simulink model "predictive_continuous_simulation_20241118_2015b"  (R2015b)
settings: Solver=ode4  SolverMode=SingleTasking  StartTime=0.0  StopTime=Tend  FixedStep=Ts  MaxStep=Ts  MinStep=Ts  RelTol=1e-3
values from neighbouring files (symbols this model uses):
  gamma = 2    [code_simu.m]    (also in code_simu_continuous_simplified.m = 100000; matlab.mat = 1000)
  sigma = 10    [code_simu.m]    (also in code_simu_continuous_simplified.m = 0.01; matlab.mat = 100)
undefined symbols (not defined in the file or in its folder): ae, Afp, As, bap_bar, bap_v, be, beta0, beta1, beta2, bfp, cap_bar, den_filter, dena0, denf, denp, exp_cap2, fn, M1, M3, M3_v_2, M4_v_2, M_bar, num_filter, numa0, numf, nump, Pf, r, setpoint, setpoint_time, sin_f, T, T_gairan, Tf, Tf_n, Tf_n_vec, Tref, Ts, tstf_vec, v_max, YM
(part 1 of 2)
settings Model: Creator=IDS_PC  LastModifiedBy=IDS_PC
settings DataIOCC: LimitDataPoints=off
settings DebuggingCC: SolverPrmCheckMsg=warning  AllowSymbolicDim=on  StateNameClashWarn=warning  SFUnexpectedBacktrackingDiag=error  SFNoUnconditionalDefaultTransitionDiag=error
settings ModelReferenceCC: PropagateSignalLabelsOutOfModel=on
settings SFSimCC: SimUseLocalCustomCode=on
settings RTWCC: RTWUseLocalCustomCode=on
settings GRTTargetCC: TargetLangStandard=C99 (ISO)
settings ConfigComp: CovMetricSettings=dwe  CovSaveCumulativeToWorkspaceVar=off  CovSaveSingleToWorkspaceVar=off  CovModelRefEnable=Off  CovExternalEMLEnable=on

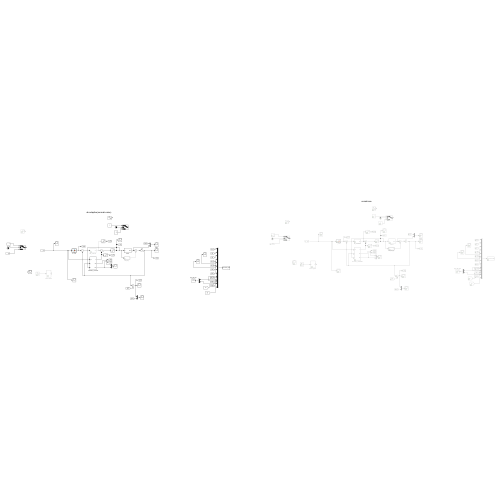
[thumbnail: Simulink's stored preview of the top-level diagram]
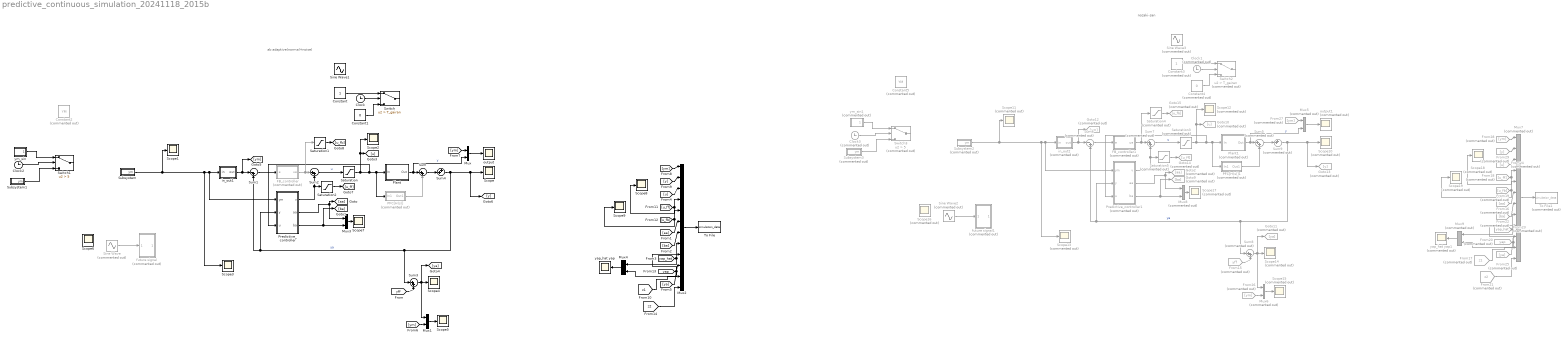
== system predictive_continuous_simulation_20241118_2015b ==
  note: ab adaptive(normal+noise)
  note: nozaki-san
  Clock : Clock
  Clock1 : Clock  Commented=on
  Clock2 : Clock
  Clock3 : Clock  Commented=on
  Constant : Constant
  Constant1 : Constant  Value=0
  Constant2 : Constant  Commented=on  Value=YM
  Constant3 : Constant  Commented=on
  Constant4 : Constant  Commented=on  Value=0
  Constant5 : Constant  Commented=on  Value=YM
  FB_controller : Subsystem  Commented=on
  FB_controller1 : Subsystem  Commented=on
  From15 : From  Commented=on  GotoTag=yff
  From16 : From  Commented=on  GotoTag=aa
  From17 : From  Commented=on  GotoTag=z1  TagVisibility=global
  From18 : From  Commented=on  GotoTag=u_ff
  From19 : From  Commented=on  GotoTag=u_fb
  From20 : From  Commented=on  GotoTag=yap  TagVisibility=global
  From21 : From  Commented=on  GotoTag=z2  TagVisibility=global
  From22 : From  Commented=on  GotoTag=ba
  From23 : From  Commented=on  GotoTag=yap_hat  TagVisibility=global
  From24 : From  Commented=on  GotoTag=u
  From25 : From  Commented=on  GotoTag=ya
  From26 : From  Commented=on  GotoTag=ym
  From27 : From  Commented=on  GotoTag=ym
  From28 : From  Commented=on  GotoTag=ym
  From29 : From  Commented=on  GotoTag=y
  Goto10 : Goto  Commented=on  GotoTag=u
  Goto11 : Goto  Commented=on  GotoTag=ya
  Goto12 : Goto  Commented=on  GotoTag=ym
  Goto13 : Goto  Commented=on  GotoTag=y
  Goto14 : Goto  Commented=on  GotoTag=u_ff
  Goto15 : Goto  Commented=on  GotoTag=u_fb
  Goto2 : Goto  Commented=on  GotoTag=aa
  Goto9 : Goto  Commented=on  GotoTag=ba
  Mux{,1,3..4} (4 alike) : Mux  Inputs=2
  Mux2 : Mux  Inputs=12
  Mux{5..6,8..9} (4 alike) : Mux  Commented=on  Inputs=2
  Mux7 : Mux  Commented=on  Inputs=12
  PFC[H(s)] : Subsystem  Commented=on  TreatAsAtomicUnit=on
  PFC[H(s)]1 : Subsystem  Commented=on  TreatAsAtomicUnit=on
  Plant : Subsystem
  Plant1 : Subsystem  Commented=on
  Predictive_controller : Subsystem
  Predictive_controller1 : Subsystem  Commented=on
  Saturation : Saturate  UpperLimit=v_max  LowerLimit=-v_max
  Saturation1 : Saturate  UpperLimit=v_max  LowerLimit=-v_max
  Saturation2 : Saturate  UpperLimit=v_max  LowerLimit=-v_max
  Saturation3 : Saturate  Commented=on  UpperLimit=v_max  LowerLimit=-v_max
  Saturation4 : Saturate  Commented=on  UpperLimit=v_max  LowerLimit=-v_max
  Saturation5 : Saturate  Commented=on  UpperLimit=v_max  LowerLimit=-v_max
  Scope{,1..9} (10 alike) : Scope
  Scope{10..19} (10 alike) : Scope  Commented=on
  Sine Wave : Sin  Commented=on  Frequency=2*pi*fn  SampleTime=0
  Sine Wave1 : Sin  Amplitude=0.1  Frequency=2*pi*1  SampleTime=0
  Sine Wave2 : Sin  Commented=on  Frequency=2*pi*fn  SampleTime=0
  Sine Wave3 : Sin  Commented=on  Amplitude=0.1  Frequency=2*pi*1  SampleTime=0
  Subsystem : Subsystem
  Subsystem1 : Subsystem
  Subsystem2 : Subsystem  Commented=on
  Subsystem3 : Subsystem  Commented=on
  Sum : Sum  Inputs=|++
  Sum1 : Sum  Inputs=|-+
  Sum2 : Sum  Inputs=|++
  Sum3 : Sum  Inputs=|++
  Sum4 : Sum  Inputs=++|
  Sum5 : Sum  Commented=on  Inputs=|++
  Sum6 : Sum  Commented=on  Inputs=|-+
  Sum7 : Sum  Commented=on  Inputs=|++
  Sum8 : Sum  Commented=on  Inputs=|++
  Sum9 : Sum  Commented=on  Inputs=++|
  Switch : Switch  Criteria=u2 > Threshold  Threshold=T_gairan
  Switch1 : Switch  Criteria=u2 > Threshold  Threshold=5
  Switch2 : Switch  Commented=on  Criteria=u2 > Threshold  Threshold=T_gairan
  Switch3 : Switch  Commented=on  Criteria=u2 > Threshold  Threshold=5
  To File : ToFile  Filename=simulation_data
  To File1 : ToFile  Commented=on  Filename=simulation_data
  future signal : Subsystem  Commented=on
  future signal1 : Subsystem  Commented=on
  in_out1 : MATLAB Function  TreatAsAtomicUnit=on
  in_out2 : MATLAB Function  Commented=on  TreatAsAtomicUnit=on
  output : Scope
  output1 : Scope  Commented=on
  yap_hat yap : Scope
  yap_hat yap1 : Scope  Commented=on
  ym_sin : Subsystem
  ym_sin1 : Subsystem  Commented=on
  wires:
  [y] -> Mux2/2
  Mux4/1 -> yap_hat yap/1
  [ym] -> Mux/1
  [yap_hat] -> Mux4/1, Mux2/8
  Mux3/1 -> Scope7/1
  Sine Wave/1 -> future signal/1(In1)
  Constant1/1 -> Switch/3
  Constant/1 -> Switch/1
  Predictive_controller/1(v) -> Saturation2/1, Sum2/2
  [u_ff] -> Scope8/1, Mux2/4
  [u] -> Mux2/3
  [yap] -> Mux4/2, Mux2/9
  [ym] -> Mux1/2
  Saturation/1 -> [u], Scope2/1, PFC[H(s)]/1(In1), Plant/1(In), Predictive_controller/3(u)
  [ym] -> Mux2/1
  [u_fb] -> Scope9/1, Mux2/5
  Saturation1/1 -> [u_fb]
  Mux1/1 -> Scope5/1
  [aa] -> Mux2/6
  Sum3/1 -> [ya], Mux1/1, Scope4/1
  Predictive_controller/3(ba) -> Mux3/2, [ba]
  Plant/1(Out) -> Mux/2, Sum/1  "y"
  Predictive_controller/2(aa) -> [aa], Mux3/1
  Subsystem/1(ym) -> Scope1/1, Predictive_controller/1(ym), in_out1/1(in), Scope3/1
  Clock/1 -> Switch/2
  [ba] -> Mux2/7
  [yff] -> Sum3/2
  [ya] -> Mux2/10
  Sum4/1 -> [y], Scope/1, Predictive_controller/2(y), Sum1/2, Sum3/1  "ya"
  Mux/1 -> output/1
  Mux2/1 -> To File/1
  Sum1/1 -> FB_controller/1(e)
  Sum2/1 -> Saturation/1  "u"
  Saturation2/1 -> [u_ff]
  FB_controller/1(ue) -> Saturation1/1, Sum2/1
  PFC[H(s)]/1(Out1) -> Sum/2
  Sum/1 -> Sum4/2
  in_out1/1(out) -> [ym], Sum1/1
  Clock2/1 -> Switch1/2
  ym_sin/1(Out1) -> Switch1/1
  Subsystem1/1(ym) -> Switch1/3
  [z1] -> Mux2/11
  [z2] -> Mux2/12
  From21/1 -> Mux7/12
  Subsystem3/1(ym) -> Switch3/3
  Saturation4/1 -> Goto15/1
  From25/1 -> Mux7/10
  Mux8/1 -> Scope17/1
  From20/1 -> Mux9/2, Mux7/9
  ym_sin1/1(Out1) -> Switch3/1
  From22/1 -> Mux7/7
  in_out2/1(out) -> Goto12/1, Sum6/1
  FB_controller1/1(ue) -> Saturation4/1, Sum7/1
  Predictive_controller1/1(v) -> Saturation5/1, Sum7/2
  Saturation5/1 -> Goto14/1
  Clock3/1 -> Switch3/2
  Sum7/1 -> Saturation3/1  "u"
  Plant1/1(Out) -> Mux5/2, Sum5/1  "y"
  From29/1 -> Mux7/2
  Sum6/1 -> FB_controller1/1(e)
  Mux5/1 -> output1/1
  Mux6/1 -> Scope15/1
  PFC[H(s)]1/1(Out1) -> Sum5/2
  From27/1 -> Mux5/1
  Subsystem2/1(ym) -> Scope11/1, Predictive_controller1/1(ym), in_out2/1(in), Scope13/1
  From18/1 -> Scope18/1, Mux7/4
  Clock1/1 -> Switch2/2
  Sum8/1 -> Goto11/1, Mux6/1, Scope14/1
  Saturation3/1 -> Goto10/1, Scope12/1, PFC[H(s)]1/1(In1), Plant1/1(In), Predictive_controller1/3(u)
  Constant3/1 -> Switch2/1
  Predictive_controller1/2(aa) -> Goto2/1, Mux8/1
  From19/1 -> Scope19/1, Mux7/5
  Sum9/1 -> Goto13/1, Scope10/1, Predictive_controller1/2(y), Sum6/2, Sum8/1  "ya"
  From24/1 -> Mux7/3
  From15/1 -> Sum8/2
  Mux7/1 -> To File1/1
  From16/1 -> Mux7/6
  From23/1 -> Mux9/1, Mux7/8
  From17/1 -> Mux7/11
  Predictive_controller1/3(ba) -> Mux8/2, Goto9/1
  From28/1 -> Mux7/1
  Sum5/1 -> Sum9/2
  From26/1 -> Mux6/2
  Mux9/1 -> yap_hat yap1/1
  Sine Wave2/1 -> future signal1/1(In1)
  Constant4/1 -> Switch2/3

== system predictive_continuous_simulation_20241118_2015b/FB_controller ==
  e : Inport
  FB_controller : Subsystem
  PFC : TransferFcn  Numerator=numa0  Denominator=dena0
  Scope : Scope
  Sum : Sum  Inputs=|++
  ue : Outport
  tag scope: yff=global
  wires:
  e/1 -> Sum/1
  PFC/1 -> [yff], Scope/1
  Sum/1 -> FB_controller/1(eaf)
  FB_controller/1(ue) -> ue/1
  ? -> PFC/1

== system predictive_continuous_simulation_20241118_2015b/FB_controller1 ==
  e : Inport
  FB_controller : Subsystem
  PFC : TransferFcn  Numerator=numa0  Denominator=dena0
  Scope : Scope
  Sum : Sum  Inputs=|++
  ue : Outport
  tag scope: yff=global
  wires:
  e/1 -> Sum/1
  PFC/1 -> [yff], Scope/1
  Sum/1 -> FB_controller/1(eaf)
  FB_controller/1(ue) -> ue/1
  ? -> PFC/1

== system predictive_continuous_simulation_20241118_2015b/PFC[H(s)] ==
  In1 : Inport
  F(s) : TransferFcn  Numerator=numf  Denominator=denf
  G0(s) : TransferFcn  Numerator=numa0  Denominator=dena0
  Sum : Sum  Inputs=|+-
  Sum1 : Sum  Inputs=|++
  Transport Delay : TransportDelay  DelayTime=T
  Out1 : Outport
  wires:
  In1/1 -> F(s)/1, Sum/1, Transport Delay/1
  G0(s)/1 -> Sum1/1
  Transport Delay/1 -> Sum/2
  Sum/1 -> G0(s)/1
  Sum1/1 -> Out1/1
  F(s)/1 -> Sum1/2

== system predictive_continuous_simulation_20241118_2015b/PFC[H(s)]1 ==
  In1 : Inport
  F(s) : TransferFcn  Numerator=numf  Denominator=denf
  G0(s) : TransferFcn  Numerator=numa0  Denominator=dena0
  Sum : Sum  Inputs=|+-
  Sum1 : Sum  Inputs=|++
  Transport Delay : TransportDelay  DelayTime=T
  Out1 : Outport
  wires:
  In1/1 -> F(s)/1, Sum/1, Transport Delay/1
  G0(s)/1 -> Sum1/1
  Transport Delay/1 -> Sum/2
  Sum/1 -> G0(s)/1
  Sum1/1 -> Out1/1
  F(s)/1 -> Sum1/2

== system predictive_continuous_simulation_20241118_2015b/Plant ==
  In : Inport
  Transfer Fcn : TransferFcn  Numerator=nump  Denominator=denp
  Transport Delay : TransportDelay  DelayTime=T
  Out : Outport
  wires:
  Transfer Fcn/1 -> Out/1
  In/1 -> Transport Delay/1
  Transport Delay/1 -> Transfer Fcn/1

== system predictive_continuous_simulation_20241118_2015b/Plant1 ==
  In : Inport
  Transfer Fcn : TransferFcn  Numerator=nump  Denominator=denp
  Transport Delay : TransportDelay  DelayTime=T
  Out : Outport
  wires:
  Transfer Fcn/1 -> Out/1
  In/1 -> Transport Delay/1
  Transport Delay/1 -> Transfer Fcn/1

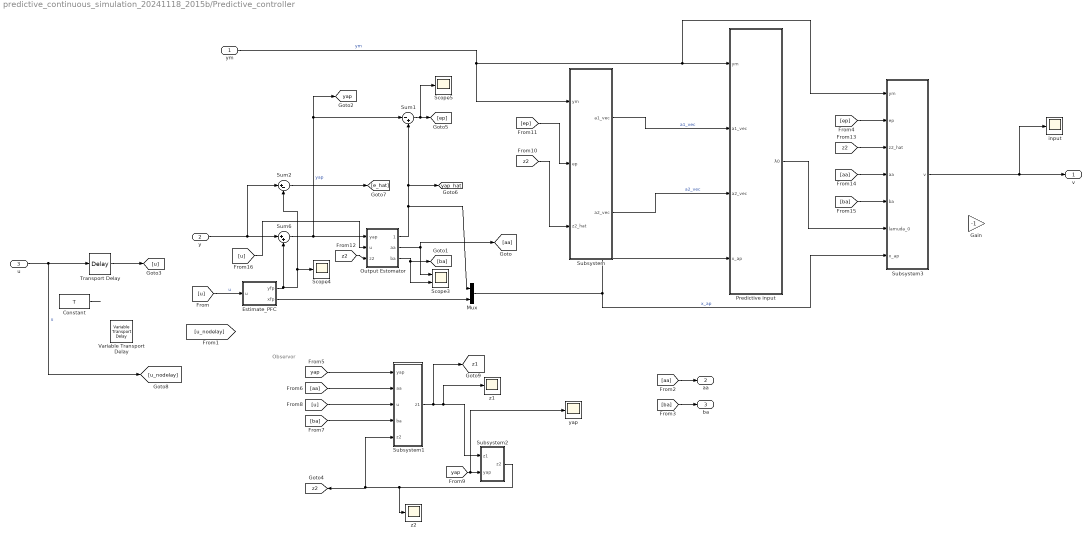
== system predictive_continuous_simulation_20241118_2015b/Predictive_controller ==
  note: Observor
  ym : Inport
  y : Inport  Port=2
  u : Inport  Port=3
  Constant : Constant  Value=T
  Estimate_PFC : Subsystem
  Gain : Gain  Gain=-1
  Mux : Mux  Inputs=2
  Output Estomator : Subsystem
  Predictive input : Subsystem
  Scope3 : Scope  NumInputPorts=2
  Scope4 : Scope
  Scope5 : Scope
  Subsystem : Subsystem
  Subsystem1 : Subsystem
  Subsystem2 : Subsystem
  Subsystem3 : Subsystem
  Sum1 : Sum  Inputs=|-+
  Sum2 : Sum  Inputs=|+-
  Sum6 : Sum  Inputs=|++
  Transport Delay : TransportDelay  DelayTime=T
  Variable Transport Delay : VariableTransportDelay  MaximumDelay=10
  input : Scope
  yap : Scope
  z1 : Scope
  z2 : Scope
  v : Outport
  aa : Outport  Port=2
  ba : Outport  Port=3
  tag scope: yap=global, yap_hat=global, z1=global, z2=global
  wires:
  y/1 -> Sum2/1, Sum6/1
  Estimate_PFC/1(yfp) -> Scope4/1, Sum2/2, Sum6/2
  Sum6/1 -> Sum1/1, [yap], Output Estomator/1(yap)  "yap"
  Output Estomator/1(yap_hat) -> Mux/1, [yap_hat], Sum1/2
  Estimate_PFC/2(xfp) -> Mux/2
  ym/1 -> Subsystem/1(ym), Subsystem3/1(ym), Predictive input/1(ym)  "ym"
  Mux/1 -> Predictive input/4(x_ap), Subsystem3/7(x_ap)  "x_ap"
  Subsystem/2(a2_vec) -> Predictive input/3(a2_vec)  "a2_vec"
  Subsystem/1(a1_vec) -> Predictive input/2(a1_vec)  "a1_vec"
  u/1 -> Transport Delay/1, [u_nodelay]  "u"
  [z2] -> Subsystem/3(z2_hat)
  Output Estomator/2(aa) -> [aa], Scope3/1
  Output Estomator/3(ba) -> [ba], Scope3/2
  [aa] -> aa/1
  [ba] -> ba/1
  [yap] -> Subsystem1/1(yap)
  [aa] -> Subsystem1/2(aa)
  [u] -> Subsystem1/3(u)
  [ba] -> Subsystem1/4("ba ")
  Subsystem2/1(z2) -> z2/1, Subsystem1/5(z2), [z2]
  Sum1/1 -> Scope5/1, [ep]
  [ep] -> Subsystem/2(ep)
  [z2] -> Output Estomator/3("z2 ")
  Sum2/1 -> [e_hat]
  Predictive input/1(λ0) -> Subsystem3/6("lamuda_0 ")
  [ba] -> Subsystem3/5(ba)
  [aa] -> Subsystem3/4(aa)
  [z2] -> Subsystem3/3(z2_hat)
  [ep] -> Subsystem3/2(ep)
  [u] -> Estimate_PFC/1(u)  "u"
  [u] -> Output Estomator/2(u)
  Constant/1 -> ?
  [yap] -> yap/1, Subsystem2/2(yap)
  Transport Delay/1 -> [u]
  Subsystem3/1(v) -> input/1, v/1
  Subsystem1/1(z1) -> [z1], z1/1, Subsystem2/1(z1)

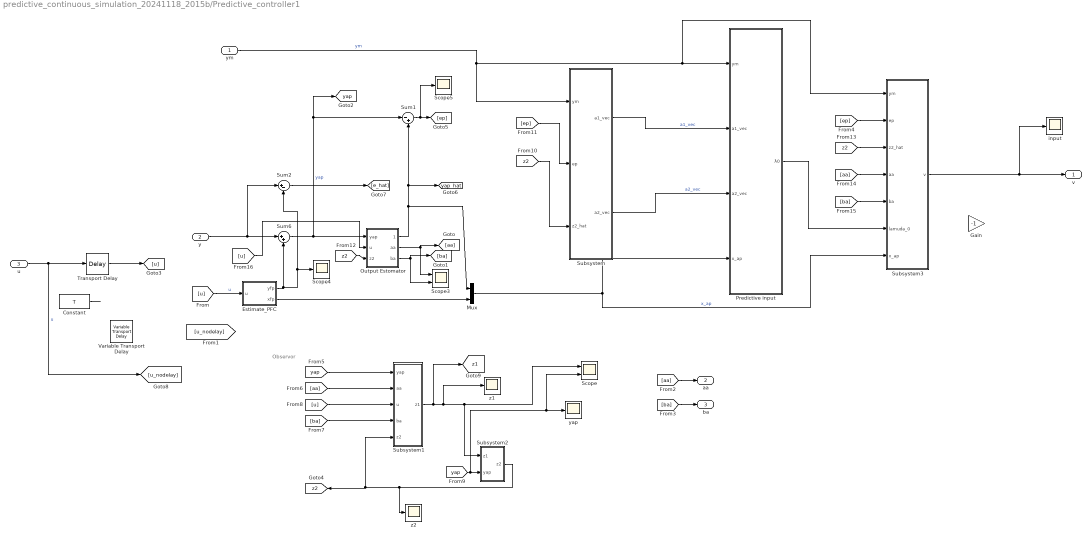
== system predictive_continuous_simulation_20241118_2015b/Predictive_controller1 ==
  note: Observor
  ym : Inport
  y : Inport  Port=2
  u : Inport  Port=3
  Constant : Constant  Value=T
  Estimate_PFC : Subsystem
  Gain : Gain  Gain=-1
  Mux : Mux  Inputs=2
  Output Estomator : Subsystem
  Predictive input : Subsystem
  Scope : Scope  NumInputPorts=2
  Scope3 : Scope  NumInputPorts=2
  Scope4 : Scope
  Scope5 : Scope
  Subsystem : Subsystem
  Subsystem1 : Subsystem
  Subsystem2 : Subsystem
  Subsystem3 : Subsystem
  Sum1 : Sum  Inputs=|-+
  Sum2 : Sum  Inputs=|+-
  Sum6 : Sum  Inputs=|++
  Transport Delay : TransportDelay  DelayTime=T
  Variable Transport Delay : VariableTransportDelay  MaximumDelay=10
  input : Scope
  yap : Scope
  z1 : Scope
  z2 : Scope
  v : Outport
  aa : Outport  Port=2
  ba : Outport  Port=3
  tag scope: yap=global, yap_hat=global, z1=global, z2=global
  wires:
  y/1 -> Sum2/1, Sum6/1
  Estimate_PFC/1(yfp) -> Scope4/1, Sum2/2, Sum6/2
  Sum6/1 -> Sum1/1, [yap], Output Estomator/1(yap)  "yap"
  Output Estomator/1(yap_hat) -> Mux/1, [yap_hat], Sum1/2
  Estimate_PFC/2(xfp) -> Mux/2
  ym/1 -> Subsystem/1(ym), Subsystem3/1(ym), Predictive input/1(ym)  "ym"
  Mux/1 -> Predictive input/4(x_ap), Subsystem3/7(x_ap)  "x_ap"
  Subsystem/2(a2_vec) -> Predictive input/3(a2_vec)  "a2_vec"
  Subsystem/1(a1_vec) -> Predictive input/2(a1_vec)  "a1_vec"
  u/1 -> Transport Delay/1, [u_nodelay]  "u"
  [z2] -> Subsystem/3(z2_hat)
  Output Estomator/2(aa) -> [aa], Scope3/1
  Output Estomator/3(ba) -> [ba], Scope3/2
  [aa] -> aa/1
  [ba] -> ba/1
  [yap] -> Subsystem1/1(yap)
  [aa] -> Subsystem1/2(aa)
  [u] -> Subsystem1/3(u)
  [ba] -> Subsystem1/4("ba ")
  Subsystem2/1(z2) -> z2/1, Subsystem1/5(z2), [z2]
  Sum1/1 -> Scope5/1, [ep]
  [ep] -> Subsystem/2(ep)
  [z2] -> Output Estomator/3("z2 ")
  Sum2/1 -> [e_hat]
  Predictive input/1(λ0) -> Subsystem3/6("lamuda_0 ")
  [ba] -> Subsystem3/5(ba)
  [aa] -> Subsystem3/4(aa)
  [z2] -> Subsystem3/3(z2_hat)
  [ep] -> Subsystem3/2(ep)
  [u] -> Estimate_PFC/1(u)  "u"
  [u] -> Output Estomator/2(u)
  Constant/1 -> ?
  [yap] -> Scope/2, yap/1, Subsystem2/2(yap)
  Subsystem3/1(v) -> input/1, v/1
  Subsystem1/1(z1) -> Scope/1, Subsystem2/1(z1), z1/1, [z1]
  Transport Delay/1 -> [u]

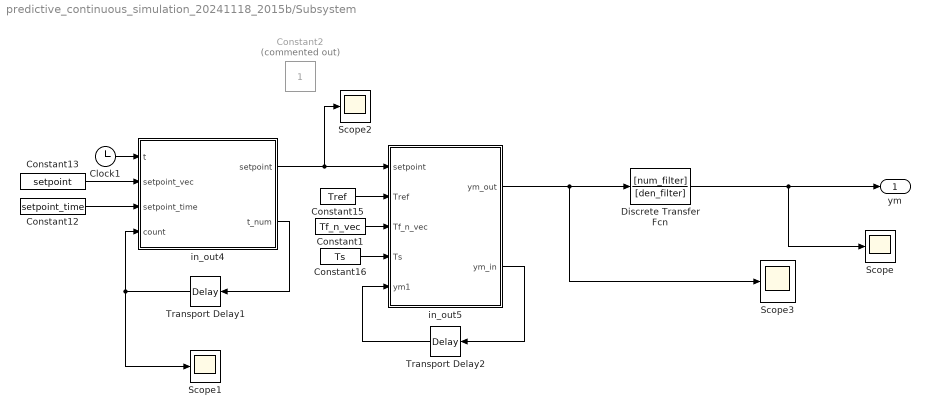
== system predictive_continuous_simulation_20241118_2015b/Subsystem ==
  Clock1 : Clock
  Constant1 : Constant  Value=Tf_n_vec
  Constant12 : Constant  Value=setpoint_time
  Constant13 : Constant  Value=setpoint
  Constant15 : Constant  Value=Tref
  Constant16 : Constant  Value=Ts
  Constant2 : Constant  Commented=on
  Discrete Transfer Fcn : DiscreteTransferFcn  Numerator=[num_filter]  Denominator=[den_filter]
  Scope{,1..3} (4 alike) : Scope
  Transport Delay1 : TransportDelay  DelayTime=Ts  InitialOutput=1
  Transport Delay2 : TransportDelay  DelayTime=Ts
  in_out4 : MATLAB Function  TreatAsAtomicUnit=on
  in_out5 : MATLAB Function  TreatAsAtomicUnit=on
  ym : Outport
  wires:
  Constant12/1 -> in_out4/3(setpoint_time)
  in_out4/2(t_num) -> Transport Delay1/1
  Transport Delay1/1 -> Scope1/1, in_out4/4(count)
  Constant13/1 -> in_out4/2(setpoint_vec)
  Constant15/1 -> in_out5/2(Tref)
  Constant16/1 -> in_out5/4(Ts)
  Transport Delay2/1 -> in_out5/5(ym1)
  in_out5/2(ym_in) -> Transport Delay2/1
  Constant1/1 -> in_out5/3(Tf_n_vec)
  Clock1/1 -> in_out4/1(t)
  in_out4/1(setpoint) -> Scope2/1, in_out5/1(setpoint)
  in_out5/1(ym_out) -> Discrete Transfer Fcn/1, Scope3/1
  Discrete Transfer Fcn/1 -> Scope/1, ym/1

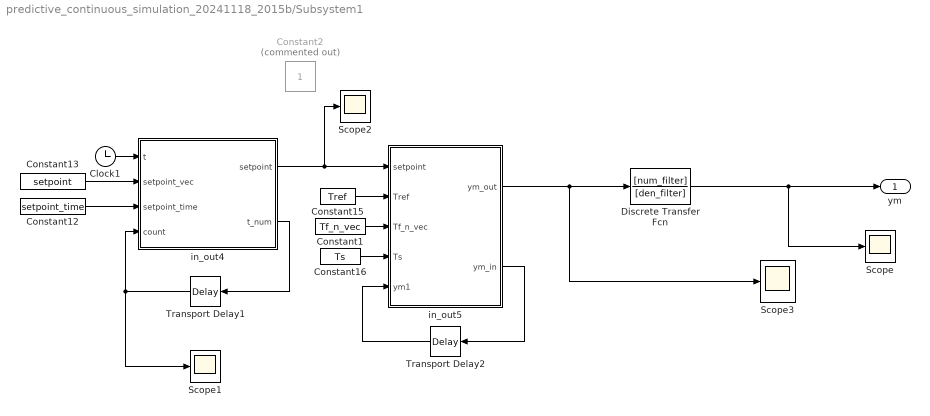
== system predictive_continuous_simulation_20241118_2015b/Subsystem1 ==
  Clock1 : Clock
  Constant1 : Constant  Value=Tf_n_vec
  Constant12 : Constant  Value=setpoint_time
  Constant13 : Constant  Value=setpoint
  Constant15 : Constant  Value=Tref
  Constant16 : Constant  Value=Ts
  Constant2 : Constant  Commented=on
  Discrete Transfer Fcn : DiscreteTransferFcn  Numerator=[num_filter]  Denominator=[den_filter]
  Scope{,1..3} (4 alike) : Scope
  Transport Delay1 : TransportDelay  DelayTime=Ts  InitialOutput=1
  Transport Delay2 : TransportDelay  DelayTime=Ts
  in_out4 : MATLAB Function  TreatAsAtomicUnit=on
  in_out5 : MATLAB Function  TreatAsAtomicUnit=on
  ym : Outport
  wires:
  Discrete Transfer Fcn/1 -> ym/1, Scope/1
  in_out5/1(ym_out) -> Scope3/1, Discrete Transfer Fcn/1
  in_out4/1(setpoint) -> in_out5/1(setpoint), Scope2/1
  Clock1/1 -> in_out4/1(t)
  Constant1/1 -> in_out5/3(Tf_n_vec)
  in_out5/2(ym_in) -> Transport Delay2/1
  Transport Delay2/1 -> in_out5/5(ym1)
  Constant16/1 -> in_out5/4(Ts)
  Constant15/1 -> in_out5/2(Tref)
  Constant13/1 -> in_out4/2(setpoint_vec)
  Transport Delay1/1 -> in_out4/4(count), Scope1/1
  in_out4/2(t_num) -> Transport Delay1/1
  Constant12/1 -> in_out4/3(setpoint_time)

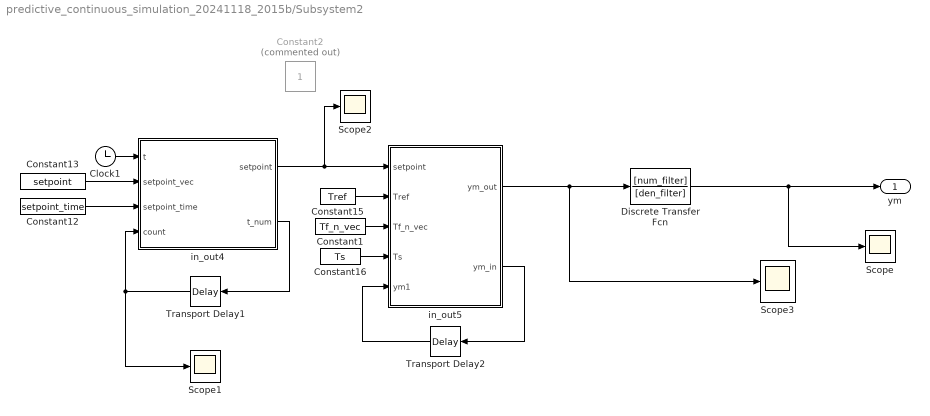
== system predictive_continuous_simulation_20241118_2015b/Subsystem2 ==
  Clock1 : Clock
  Constant1 : Constant  Value=Tf_n_vec
  Constant12 : Constant  Value=setpoint_time
  Constant13 : Constant  Value=setpoint
  Constant15 : Constant  Value=Tref
  Constant16 : Constant  Value=Ts
  Constant2 : Constant  Commented=on
  Discrete Transfer Fcn : DiscreteTransferFcn  Numerator=[num_filter]  Denominator=[den_filter]
  Scope{,1..3} (4 alike) : Scope
  Transport Delay1 : TransportDelay  DelayTime=Ts  InitialOutput=1
  Transport Delay2 : TransportDelay  DelayTime=Ts
  in_out4 : MATLAB Function  TreatAsAtomicUnit=on
  in_out5 : MATLAB Function  TreatAsAtomicUnit=on
  ym : Outport
  wires:
  Constant12/1 -> in_out4/3(setpoint_time)
  in_out4/2(t_num) -> Transport Delay1/1
  Transport Delay1/1 -> Scope1/1, in_out4/4(count)
  Constant13/1 -> in_out4/2(setpoint_vec)
  Constant15/1 -> in_out5/2(Tref)
  Constant16/1 -> in_out5/4(Ts)
  Transport Delay2/1 -> in_out5/5(ym1)
  in_out5/2(ym_in) -> Transport Delay2/1
  Constant1/1 -> in_out5/3(Tf_n_vec)
  Clock1/1 -> in_out4/1(t)
  in_out4/1(setpoint) -> Scope2/1, in_out5/1(setpoint)
  in_out5/1(ym_out) -> Discrete Transfer Fcn/1, Scope3/1
  Discrete Transfer Fcn/1 -> Scope/1, ym/1

== system predictive_continuous_simulation_20241118_2015b/Subsystem3 ==
  Clock1 : Clock
  Constant1 : Constant  Value=Tf_n_vec
  Constant12 : Constant  Value=setpoint_time
  Constant13 : Constant  Value=setpoint
  Constant15 : Constant  Value=Tref
  Constant16 : Constant  Value=Ts
  Constant2 : Constant  Commented=on
  Discrete Transfer Fcn : DiscreteTransferFcn  Numerator=[num_filter]  Denominator=[den_filter]
  Scope{,1..3} (4 alike) : Scope
  Transport Delay1 : TransportDelay  DelayTime=Ts  InitialOutput=1
  Transport Delay2 : TransportDelay  DelayTime=Ts
  in_out4 : MATLAB Function  TreatAsAtomicUnit=on
  in_out5 : MATLAB Function  TreatAsAtomicUnit=on
  ym : Outport
  wires:
  Discrete Transfer Fcn/1 -> ym/1, Scope/1
  in_out5/1(ym_out) -> Scope3/1, Discrete Transfer Fcn/1
  in_out4/1(setpoint) -> in_out5/1(setpoint), Scope2/1
  Clock1/1 -> in_out4/1(t)
  Constant1/1 -> in_out5/3(Tf_n_vec)
  in_out5/2(ym_in) -> Transport Delay2/1
  Transport Delay2/1 -> in_out5/5(ym1)
  Constant16/1 -> in_out5/4(Ts)
  Constant15/1 -> in_out5/2(Tref)
  Constant13/1 -> in_out4/2(setpoint_vec)
  Transport Delay1/1 -> in_out4/4(count), Scope1/1
  in_out4/2(t_num) -> Transport Delay1/1
  Constant12/1 -> in_out4/3(setpoint_time)

== system predictive_continuous_simulation_20241118_2015b/future signal ==
  In1 : Inport
  Constant : Constant  Value=Tf_n_vec
  Constant1 : Constant  Value=0
  Constant2 : Constant
  MATLAB Function : MATLAB Function  TreatAsAtomicUnit=on
  Switch : Switch  Criteria=u2 > Threshold  Threshold=0.5
  Transport Delay1 : TransportDelay  DelayTime=Ts
  Transport Delay2 : TransportDelay  DelayTime=Ts*Tf_n
  Out1 : Outport
  wires:
  In1/1 -> MATLAB Function/1(u)
  Transport Delay1/1 -> MATLAB Function/3(u_in)
  MATLAB Function/1(ym) -> Switch/1, Transport Delay1/1
  Constant/1 -> MATLAB Function/2(Tf_n_vec)
  Constant1/1 -> Switch/3
  Constant2/1 -> Transport Delay2/1
  Transport Delay2/1 -> Switch/2
  Switch/1 -> Out1/1

== system predictive_continuous_simulation_20241118_2015b/future signal1 ==
  In1 : Inport
  Constant : Constant  Value=Tf_n_vec
  Constant1 : Constant  Value=0
  Constant2 : Constant
  MATLAB Function : MATLAB Function  TreatAsAtomicUnit=on
  Switch : Switch  Criteria=u2 > Threshold  Threshold=0.5
  Transport Delay1 : TransportDelay  DelayTime=Ts
  Transport Delay2 : TransportDelay  DelayTime=Ts*Tf_n
  Out1 : Outport
  wires:
  In1/1 -> MATLAB Function/1(u)
  Transport Delay1/1 -> MATLAB Function/3(u_in)
  MATLAB Function/1(ym) -> Switch/1, Transport Delay1/1
  Constant/1 -> MATLAB Function/2(Tf_n_vec)
  Constant1/1 -> Switch/3
  Constant2/1 -> Transport Delay2/1
  Transport Delay2/1 -> Switch/2
  Switch/1 -> Out1/1

== system predictive_continuous_simulation_20241118_2015b/ym_sin ==
  Constant1 : Constant  Value=sin_f
  Constant2 : Constant  Value=Tf_n_vec
  Constant3 : Constant  Value=Ts
  Constant4 : Constant  Value=Ts
  MATLAB Function : MATLAB Function  TreatAsAtomicUnit=on
  Product : Product
  Scope : Scope
  Scope1 : Scope
  Step : Step  Time=Ts  SampleTime=0
  Sum : Sum  Inputs=|++
  Transport Delay : TransportDelay  DelayTime=Ts
  Transport Delay1 : TransportDelay  DelayTime=5
  Out1 : Outport
  wires:
  Product/1 -> Sum/1
  MATLAB Function/1(ym) -> Transport Delay1/1
  Constant2/1 -> MATLAB Function/1(Tf_n_vec)
  Constant3/1 -> MATLAB Function/3(Ts)
  Constant1/1 -> MATLAB Function/4(omega_sin)
  Constant4/1 -> Product/1
  Step/1 -> Product/2
  Sum/1 -> Scope1/1, Transport Delay/1, MATLAB Function/2(t)
  Transport Delay/1 -> Sum/2
  Transport Delay1/1 -> Scope/1, Out1/1

== system predictive_continuous_simulation_20241118_2015b/ym_sin1 ==
  Constant1 : Constant  Value=sin_f
  Constant2 : Constant  Value=Tf_n_vec
  Constant3 : Constant  Value=Ts
  Constant4 : Constant  Value=Ts
  MATLAB Function : MATLAB Function  TreatAsAtomicUnit=on
  Product : Product
  Scope : Scope
  Scope1 : Scope
  Step : Step  Time=Ts  SampleTime=0
  Sum : Sum  Inputs=|++
  Transport Delay : TransportDelay  DelayTime=Ts
  Transport Delay1 : TransportDelay  DelayTime=5
  Out1 : Outport
  wires:
  Product/1 -> Sum/1
  MATLAB Function/1(ym) -> Transport Delay1/1
  Constant2/1 -> MATLAB Function/1(Tf_n_vec)
  Constant3/1 -> MATLAB Function/3(Ts)
  Constant1/1 -> MATLAB Function/4(omega_sin)
  Constant4/1 -> Product/1
  Step/1 -> Product/2
  Sum/1 -> Scope1/1, Transport Delay/1, MATLAB Function/2(t)
  Transport Delay/1 -> Sum/2
  Transport Delay1/1 -> Scope/1, Out1/1

== system predictive_continuous_simulation_20241118_2015b/FB_controller/FB_controller ==
  eaf : Inport
  Gain : Gain  Gain=-1
  Integrator : Integrator
  Math Function : Math  Operator=square  SaturateOnIntegerOverflow=on
  Product : Product
  Product1 : Product
  Product2 : Product
  Scope : Scope
  Sum1 : Sum  Inputs=|++
  To Workspace : ToWorkspace  VariableName=theta_vec  SampleTime=-1
  γ : Constant  Value=gamma
  σ : Constant  Value=sigma
  ue : Outport
  wires:
  Math Function/1 -> Product1/1
  γ/1 -> Product1/2
  eaf/1 -> Product/1, Math Function/1
  Product1/1 -> Sum1/1
  Product2/1 -> Sum1/2
  Sum1/1 -> Integrator/1
  σ/1 -> Product2/1
  Integrator/1 -> To Workspace/1, Scope/1, Gain/1, Product2/2  "θ"
  Gain/1 -> Product/2
  Product/1 -> ue/1

== system predictive_continuous_simulation_20241118_2015b/FB_controller1/FB_controller ==
  eaf : Inport
  Gain : Gain  Gain=-1
  Integrator : Integrator
  Math Function : Math  Operator=square  SaturateOnIntegerOverflow=on
  Product : Product
  Product1 : Product
  Product2 : Product
  Scope : Scope
  Sum1 : Sum  Inputs=|++
  To Workspace : ToWorkspace  VariableName=theta_vec  SampleTime=-1
  γ : Constant  Value=gamma
  σ : Constant  Value=sigma
  ue : Outport
  wires:
  Math Function/1 -> Product1/1
  γ/1 -> Product1/2
  eaf/1 -> Product/1, Math Function/1
  Product1/1 -> Sum1/1
  Product2/1 -> Sum1/2
  Sum1/1 -> Integrator/1
  σ/1 -> Product2/1
  Integrator/1 -> To Workspace/1, Scope/1, Gain/1, Product2/2  "θ"
  Gain/1 -> Product/2
  Product/1 -> ue/1

== system predictive_continuous_simulation_20241118_2015b/Predictive_controller/Estimate_PFC ==
  u : Inport
  Gain : Gain  Gain=bfp  Multiplication=Matrix(K*u)
  Gain1 : Gain  Gain=Afp  Multiplication=Matrix(K*u) (u vector)
  Gain2 : Gain  Gain=cfp.'  Multiplication=Matrix(K*u) (u vector)
  Integrator : Integrator
  Scope : Scope
  Sum2 : Sum  Inputs=|++
  yfp : Outport
  xfp : Outport  Port=2
  wires:
  u/1 -> Gain/1
  Sum2/1 -> Integrator/1
  Gain/1 -> Sum2/1  "b_fp*u"
  Integrator/1 -> xfp/1, Gain2/1, Gain1/1  "x_fp"
  Gain1/1 -> Sum2/2
  Gain2/1 -> Scope/1, yfp/1

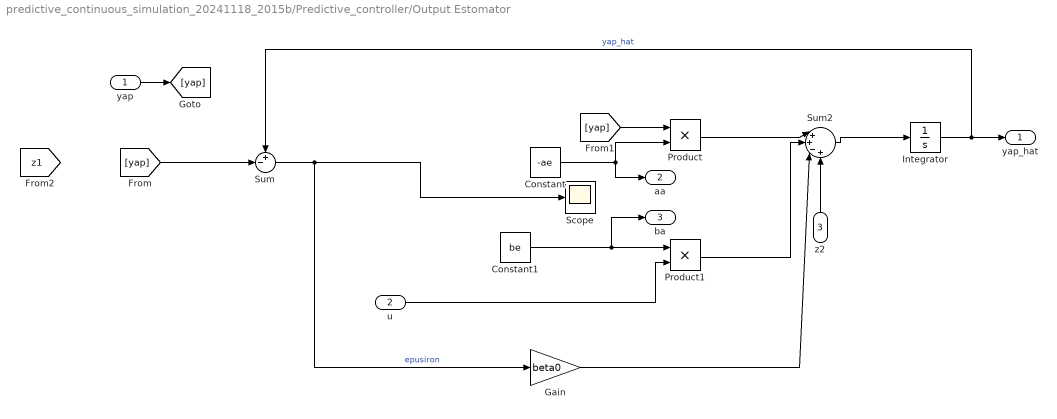
== system predictive_continuous_simulation_20241118_2015b/Predictive_controller/Output Estomator ==
  yap : Inport
  u : Inport  Port=2
  "z2 " : Inport  Port=3
  Constant : Constant  Value=-ae
  Constant1 : Constant  Value=be
  Gain : Gain  Gain=beta0
  Integrator : Integrator
  Product : Product
  Product1 : Product
  Scope : Scope
  Sum : Sum  Inputs=+-|
  Sum2 : Sum  Inputs=|++-+
  yap_hat : Outport
  aa : Outport  Port=2
  ba : Outport  Port=3
  wires:
  Sum/1 -> Gain/1, Scope/1  "epusiron"
  Product1/1 -> Sum2/2
  Sum2/1 -> Integrator/1
  Product/1 -> Sum2/1
  [yap] -> Sum/2
  u/1 -> Product1/2
  Constant/1 -> aa/1, Product/2
  Constant1/1 -> ba/1, Product1/1
  Integrator/1 -> Sum/1, yap_hat/1  "yap_hat"
  Gain/1 -> Sum2/3
  "z2 "/1 -> Sum2/4
  yap/1 -> [yap]
  [yap] -> Product/1

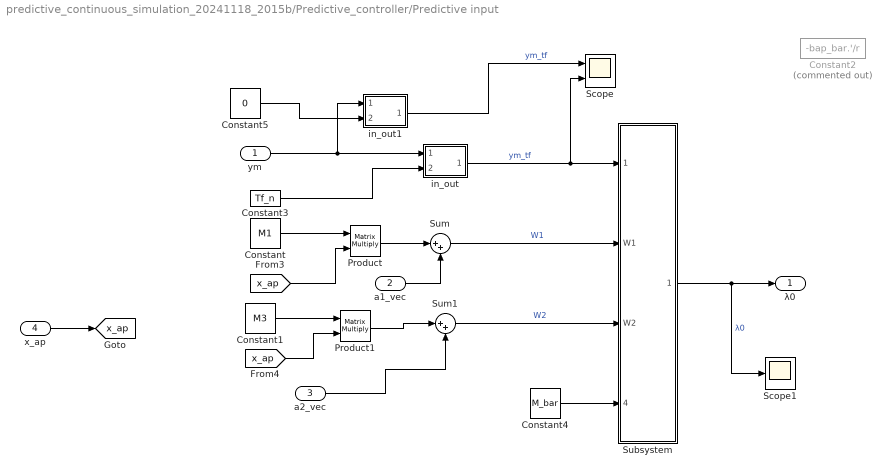
== system predictive_continuous_simulation_20241118_2015b/Predictive_controller/Predictive input ==
  ym : Inport
  a1_vec : Inport  Port=2
  a2_vec : Inport  Port=3
  x_ap : Inport  Port=4
  Constant : Constant  Value=M1
  Constant1 : Constant  Value=M3
  Constant2 : Constant  Commented=on  Value=-bap_bar.'/r  VectorParams1D=off  SampleTime=-1
  Constant3 : Constant  Value=Tf_n
  Constant4 : Constant  Value=M_bar
  Constant5 : Constant  Value=0
  Product : Product  Multiplication=Matrix(*)
  Product1 : Product  Multiplication=Matrix(*)
  Scope : Scope  NumInputPorts=2
  Scope1 : Scope
  Subsystem : Subsystem
  Sum : Sum  Inputs=|++
  Sum1 : Sum  Inputs=|++
  in_out : MATLAB Function  TreatAsAtomicUnit=on
  in_out1 : MATLAB Function  TreatAsAtomicUnit=on
  λ0 : Outport
  tag scope: x_ap=global
  wires:
  x_ap/1 -> [x_ap]
  Constant/1 -> Product/1
  [x_ap] -> Product/2
  Product/1 -> Sum/1
  a1_vec/1 -> Sum/2
  Constant1/1 -> Product1/1
  [x_ap] -> Product1/2
  Product1/1 -> Sum1/1
  a2_vec/1 -> Sum1/2
  ym/1 -> in_out1/1(ym_vec), in_out/1(ym_vec)
  in_out/1(ym_tf) -> Scope/2, Subsystem/1(ym_tf)  "ym_tf"
  Sum1/1 -> Subsystem/3(W2)  "W2"
  Sum/1 -> Subsystem/2(W1)  "W1"
  Constant3/1 -> in_out/2(Tf_n)
  Constant4/1 -> Subsystem/4(M_bar)
  Subsystem/1(lambda_0) -> Scope1/1, λ0/1  "λ0"
  Constant5/1 -> in_out1/2(Tf_n)
  in_out1/1(ym_tf) -> Scope/1  "ym_tf"

== system predictive_continuous_simulation_20241118_2015b/Predictive_controller/Subsystem ==
  ym : Inport
  ep : Inport  Port=2
  z2_hat : Inport  Port=3
  Constant : Constant  Value=cap_bar
  Constant2 : Constant  Value=beta0
  Constant3 : Constant  Value=Tf_n
  Constant4 : Constant  Value=Ts
  Constant5 : Constant  Value=Tf
  Constant6 : Constant  Value=tstf_vec
  MATLAB Function1 : MATLAB Function  TreatAsAtomicUnit=on
  a1_vec : Outport
  a2_vec : Outport  Port=2
  wires:
  ym/1 -> MATLAB Function1/1(ym)
  ep/1 -> MATLAB Function1/2(ep)
  z2_hat/1 -> MATLAB Function1/3(z2_hat)
  Constant/1 -> MATLAB Function1/4(cap_bar)
  Constant2/1 -> MATLAB Function1/5(beta0)
  MATLAB Function1/2(a2_vec) -> a2_vec/1
  MATLAB Function1/1(a1_vec) -> a1_vec/1
  Constant3/1 -> MATLAB Function1/6(Tf_n)
  Constant4/1 -> MATLAB Function1/7(Ts)
  Constant5/1 -> MATLAB Function1/8(Tf)
  Constant6/1 -> MATLAB Function1/9(tstf_vec)

== system predictive_continuous_simulation_20241118_2015b/Predictive_controller/Subsystem1 ==
  yap : Inport
  aa : Inport  Port=2
  u : Inport  Port=3
  "ba " : Inport  Port=4
  z2 : Inport  Port=5
  Gain : Gain  Gain=-beta1
  Integrator : Integrator
  Product : Product
  Product1 : Product
  Sum2 : Sum  Inputs=|++
  Sum3 : Sum  Inputs=-+|
  Sum4 : Sum  Inputs=++|
  Sum5 : Sum  Inputs=|++
  z1 : Outport
  wires:
  Sum2/1 -> Sum4/2
  u/1 -> Product1/1
  Product/1 -> Sum2/1
  yap/1 -> Sum3/1
  Sum4/1 -> Sum5/1
  Gain/1 -> Sum4/1
  Product1/1 -> Sum2/2
  Integrator/1 -> z1/1, Product/1, Sum3/2
  z2/1 -> Sum5/2
  "ba "/1 -> Product1/2
  Sum5/1 -> Integrator/1
  Sum3/1 -> Gain/1
  aa/1 -> Product/2

== system predictive_continuous_simulation_20241118_2015b/Predictive_controller/Subsystem2 ==
  z1 : Inport
  yap : Inport  Port=2
  Gain1 : Gain  Gain=-beta2
  Integrator1 : Integrator
  Sum7 : Sum  Inputs=+-|
  z2 : Outport
  wires:
  yap/1 -> Sum7/2
  Sum7/1 -> Gain1/1
  Integrator1/1 -> z2/1
  z1/1 -> Sum7/1
  Gain1/1 -> Integrator1/1

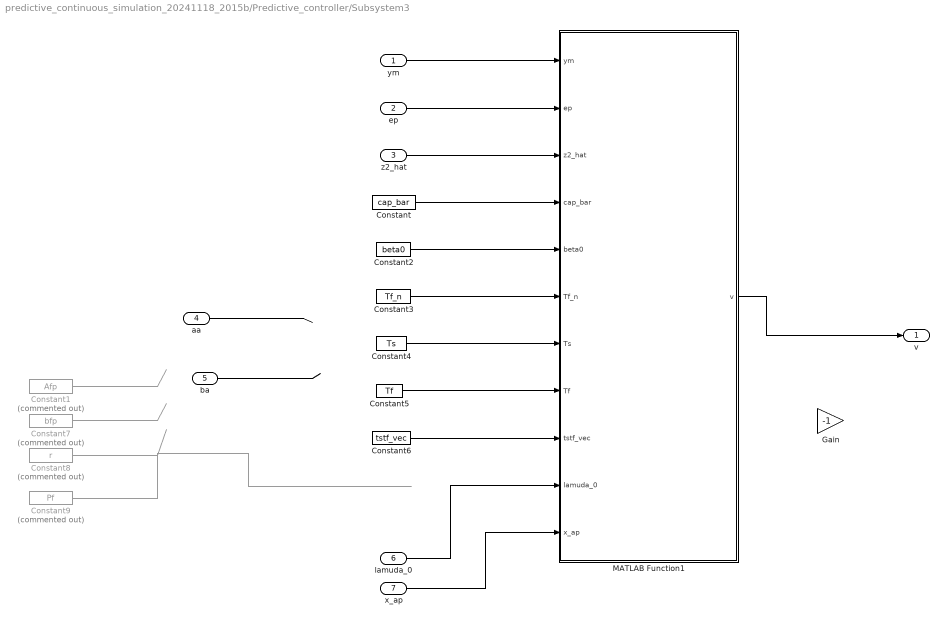
== system predictive_continuous_simulation_20241118_2015b/Predictive_controller/Subsystem3 ==
  ym : Inport
  ep : Inport  Port=2
  z2_hat : Inport  Port=3
  aa : Inport  Port=4
  ba : Inport  Port=5
  "lamuda_0 " : Inport  Port=6
  x_ap : Inport  Port=7
  Constant : Constant  Value=cap_bar
  Constant1 : Constant  Commented=on  Value=Afp
  Constant2 : Constant  Value=beta0
  Constant3 : Constant  Value=Tf_n
  Constant4 : Constant  Value=Ts
  Constant5 : Constant  Value=Tf
  Constant6 : Constant  Value=tstf_vec
  Constant7 : Constant  Commented=on  Value=bfp
  Constant8 : Constant  Commented=on  Value=r
  Constant9 : Constant  Commented=on  Value=Pf
  Gain : Gain  Gain=-1
  MATLAB Function1 : MATLAB Function  TreatAsAtomicUnit=on
      settings: MinAlgLoopOccurrences=on
  v : Outport
  wires:
  ym/1 -> MATLAB Function1/1(ym)
  ep/1 -> MATLAB Function1/2(ep)
  z2_hat/1 -> MATLAB Function1/3(z2_hat)
  Constant/1 -> MATLAB Function1/4(cap_bar)
  Constant2/1 -> MATLAB Function1/5(beta0)
  Constant3/1 -> MATLAB Function1/6(Tf_n)
  Constant4/1 -> MATLAB Function1/7(Ts)
  Constant5/1 -> MATLAB Function1/8(Tf)
  Constant6/1 -> MATLAB Function1/9(tstf_vec)
  aa/1 -> ?
  ba/1 -> ?
  Constant1/1 -> ?
  Constant7/1 -> ?
  Constant8/1 -> ?
  Constant9/1 -> ?
  "lamuda_0 "/1 -> MATLAB Function1/10(lamuda_0)
  x_ap/1 -> MATLAB Function1/11(x_ap)
  MATLAB Function1/1(v) -> v/1

== system predictive_continuous_simulation_20241118_2015b/Predictive_controller1/Estimate_PFC ==
  u : Inport
  Gain : Gain  Gain=bfp  Multiplication=Matrix(K*u)
  Gain1 : Gain  Gain=Afp  Multiplication=Matrix(K*u) (u vector)
  Gain2 : Gain  Gain=cfp.'  Multiplication=Matrix(K*u) (u vector)
  Integrator : Integrator
  Scope : Scope
  Sum2 : Sum  Inputs=|++
  yfp : Outport
  xfp : Outport  Port=2
  wires:
  u/1 -> Gain/1
  Sum2/1 -> Integrator/1
  Gain/1 -> Sum2/1  "b_fp*u"
  Integrator/1 -> xfp/1, Gain2/1, Gain1/1  "x_fp"
  Gain1/1 -> Sum2/2
  Gain2/1 -> Scope/1, yfp/1

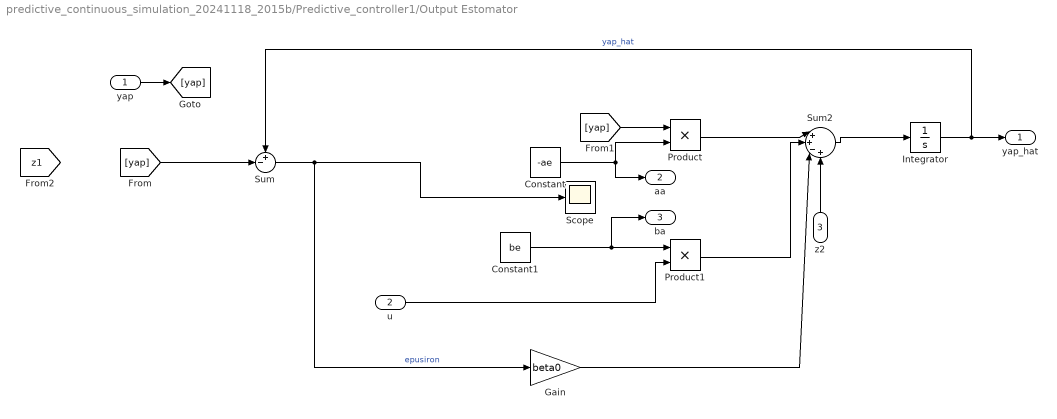
== system predictive_continuous_simulation_20241118_2015b/Predictive_controller1/Output Estomator ==
  yap : Inport
  u : Inport  Port=2
  "z2 " : Inport  Port=3
  Constant : Constant  Value=-ae
  Constant1 : Constant  Value=be
  Gain : Gain  Gain=beta0
  Integrator : Integrator
  Product : Product
  Product1 : Product
  Scope : Scope
  Sum : Sum  Inputs=+-|
  Sum2 : Sum  Inputs=|++-+
  yap_hat : Outport
  aa : Outport  Port=2
  ba : Outport  Port=3
  wires:
  Sum/1 -> Gain/1, Scope/1  "epusiron"
  Product1/1 -> Sum2/2
  Sum2/1 -> Integrator/1
  Product/1 -> Sum2/1
  [yap] -> Sum/2
  u/1 -> Product1/2
  Constant/1 -> aa/1, Product/2
  Constant1/1 -> ba/1, Product1/1
  Integrator/1 -> Sum/1, yap_hat/1  "yap_hat"
  Gain/1 -> Sum2/3
  "z2 "/1 -> Sum2/4
  yap/1 -> [yap]
  [yap] -> Product/1

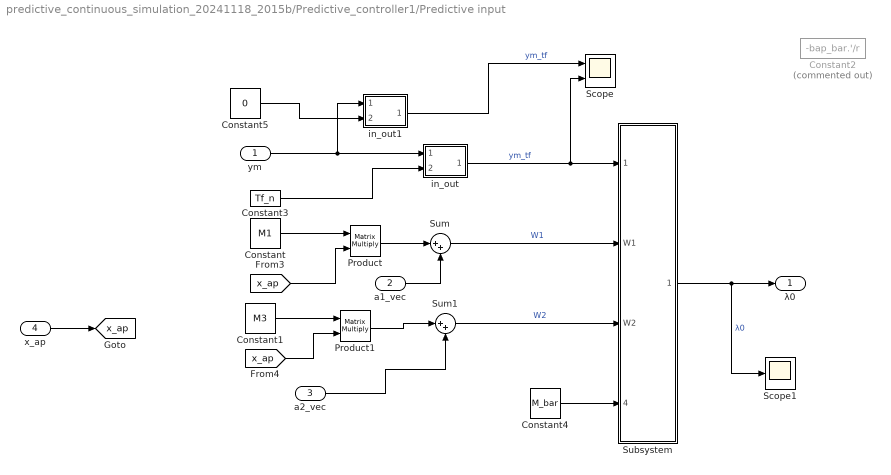
== system predictive_continuous_simulation_20241118_2015b/Predictive_controller1/Predictive input ==
  ym : Inport
  a1_vec : Inport  Port=2
  a2_vec : Inport  Port=3
  x_ap : Inport  Port=4
  Constant : Constant  Value=M1
  Constant1 : Constant  Value=M3
  Constant2 : Constant  Commented=on  Value=-bap_bar.'/r  VectorParams1D=off  SampleTime=-1
  Constant3 : Constant  Value=Tf_n
  Constant4 : Constant  Value=M_bar
  Constant5 : Constant  Value=0
  Product : Product  Multiplication=Matrix(*)
  Product1 : Product  Multiplication=Matrix(*)
  Scope : Scope  NumInputPorts=2
  Scope1 : Scope
  Subsystem : Subsystem
  Sum : Sum  Inputs=|++
  Sum1 : Sum  Inputs=|++
  in_out : MATLAB Function  TreatAsAtomicUnit=on
  in_out1 : MATLAB Function  TreatAsAtomicUnit=on
  λ0 : Outport
  tag scope: x_ap=global
  wires:
  x_ap/1 -> [x_ap]
  Constant/1 -> Product/1
  [x_ap] -> Product/2
  Product/1 -> Sum/1
  a1_vec/1 -> Sum/2
  Constant1/1 -> Product1/1
  [x_ap] -> Product1/2
  Product1/1 -> Sum1/1
  a2_vec/1 -> Sum1/2
  ym/1 -> in_out1/1(ym_vec), in_out/1(ym_vec)
  in_out/1(ym_tf) -> Scope/2, Subsystem/1(ym_tf)  "ym_tf"
  Sum1/1 -> Subsystem/3(W2)  "W2"
  Sum/1 -> Subsystem/2(W1)  "W1"
  Constant3/1 -> in_out/2(Tf_n)
  Constant4/1 -> Subsystem/4(M_bar)
  Subsystem/1(lambda_0) -> Scope1/1, λ0/1  "λ0"
  Constant5/1 -> in_out1/2(Tf_n)
  in_out1/1(ym_tf) -> Scope/1  "ym_tf"

== system predictive_continuous_simulation_20241118_2015b/Predictive_controller1/Subsystem ==
  ym : Inport
  ep : Inport  Port=2
  z2_hat : Inport  Port=3
  Constant : Constant  Value=cap_bar
  Constant2 : Constant  Value=beta0
  Constant3 : Constant  Value=Tf_n
  Constant4 : Constant  Value=Ts
  Constant5 : Constant  Value=Tf
  Constant6 : Constant  Value=tstf_vec
  MATLAB Function1 : MATLAB Function  TreatAsAtomicUnit=on
  a1_vec : Outport
  a2_vec : Outport  Port=2
  wires:
  ym/1 -> MATLAB Function1/1(ym)
  ep/1 -> MATLAB Function1/2(ep)
  z2_hat/1 -> MATLAB Function1/3(z2_hat)
  Constant/1 -> MATLAB Function1/4(cap_bar)
  Constant2/1 -> MATLAB Function1/5(beta0)
  MATLAB Function1/2(a2_vec) -> a2_vec/1
  MATLAB Function1/1(a1_vec) -> a1_vec/1
  Constant3/1 -> MATLAB Function1/6(Tf_n)
  Constant4/1 -> MATLAB Function1/7(Ts)
  Constant5/1 -> MATLAB Function1/8(Tf)
  Constant6/1 -> MATLAB Function1/9(tstf_vec)

== system predictive_continuous_simulation_20241118_2015b/Predictive_controller1/Subsystem1 ==
  yap : Inport
  aa : Inport  Port=2
  u : Inport  Port=3
  "ba " : Inport  Port=4
  z2 : Inport  Port=5
  Gain : Gain  Gain=-beta1
  Integrator : Integrator
  Product : Product
  Product1 : Product
  Sum2 : Sum  Inputs=|++
  Sum3 : Sum  Inputs=-+|
  Sum4 : Sum  Inputs=++|
  Sum5 : Sum  Inputs=|++
  z1 : Outport
  wires:
  Sum2/1 -> Sum4/2
  u/1 -> Product1/1
  Product/1 -> Sum2/1
  yap/1 -> Sum3/1
  Sum4/1 -> Sum5/1
  Gain/1 -> Sum4/1
  Product1/1 -> Sum2/2
  Integrator/1 -> z1/1, Product/1, Sum3/2
  z2/1 -> Sum5/2
  "ba "/1 -> Product1/2
  Sum5/1 -> Integrator/1
  Sum3/1 -> Gain/1
  aa/1 -> Product/2

== system predictive_continuous_simulation_20241118_2015b/Predictive_controller1/Subsystem2 ==
  z1 : Inport
  yap : Inport  Port=2
  Gain1 : Gain  Gain=-beta2
  Integrator1 : Integrator
  Sum7 : Sum  Inputs=+-|
  z2 : Outport
  wires:
  yap/1 -> Sum7/2
  Sum7/1 -> Gain1/1
  Integrator1/1 -> z2/1
  z1/1 -> Sum7/1
  Gain1/1 -> Integrator1/1

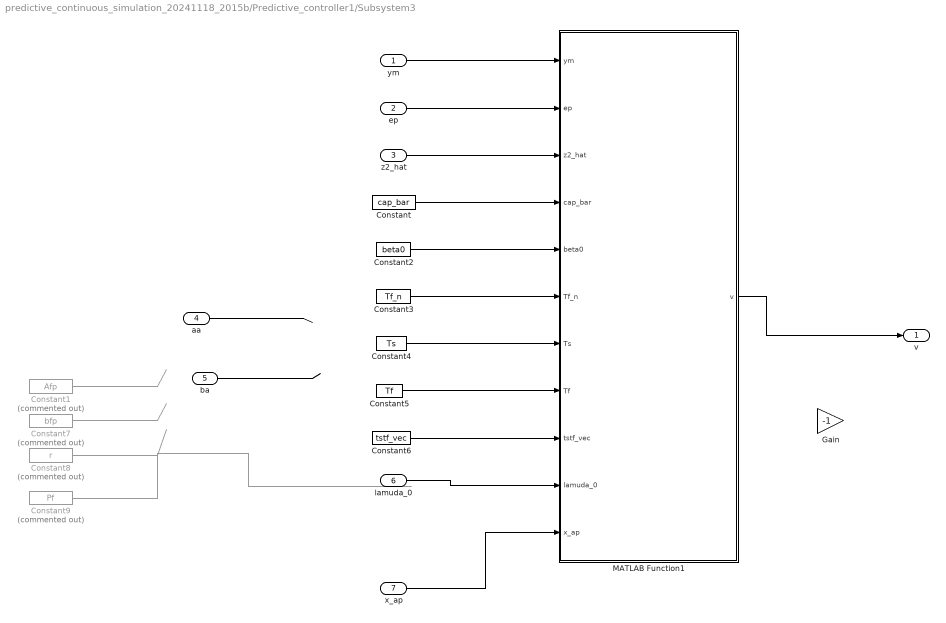
== system predictive_continuous_simulation_20241118_2015b/Predictive_controller1/Subsystem3 ==
  ym : Inport
  ep : Inport  Port=2
  z2_hat : Inport  Port=3
  aa : Inport  Port=4
  ba : Inport  Port=5
  "lamuda_0 " : Inport  Port=6
  x_ap : Inport  Port=7
  Constant : Constant  Value=cap_bar
  Constant1 : Constant  Commented=on  Value=Afp
  Constant2 : Constant  Value=beta0
  Constant3 : Constant  Value=Tf_n
  Constant4 : Constant  Value=Ts
  Constant5 : Constant  Value=Tf
  Constant6 : Constant  Value=tstf_vec
  Constant7 : Constant  Commented=on  Value=bfp
  Constant8 : Constant  Commented=on  Value=r
  Constant9 : Constant  Commented=on  Value=Pf
  Gain : Gain  Gain=-1
  MATLAB Function1 : MATLAB Function  TreatAsAtomicUnit=on
      settings: MinAlgLoopOccurrences=on
  v : Outport
  wires:
  ym/1 -> MATLAB Function1/1(ym)
  ep/1 -> MATLAB Function1/2(ep)
  z2_hat/1 -> MATLAB Function1/3(z2_hat)
  Constant/1 -> MATLAB Function1/4(cap_bar)
  Constant2/1 -> MATLAB Function1/5(beta0)
  Constant3/1 -> MATLAB Function1/6(Tf_n)
  Constant4/1 -> MATLAB Function1/7(Ts)
  Constant5/1 -> MATLAB Function1/8(Tf)
  Constant6/1 -> MATLAB Function1/9(tstf_vec)
  aa/1 -> ?
  ba/1 -> ?
  Constant1/1 -> ?
  Constant7/1 -> ?
  Constant8/1 -> ?
  Constant9/1 -> ?
  "lamuda_0 "/1 -> MATLAB Function1/10(lamuda_0)
  x_ap/1 -> MATLAB Function1/11(x_ap)
  MATLAB Function1/1(v) -> v/1

== system predictive_continuous_simulation_20241118_2015b/Predictive_controller/Predictive input/Subsystem ==
  ym_tf : Inport
  W1 : Inport  Port=2
  W2 : Inport  Port=3
  M_bar : Inport  Port=4
  Constant : Constant  Value=Pf
  Constant1 : Constant  Value=cap_bar
  MATLAB Function : MATLAB Function  TreatAsAtomicUnit=on
  lambda_0 : Outport
  wires:
  ym_tf/1 -> MATLAB Function/1(ym_tf)
  W1/1 -> MATLAB Function/2(W1)
  W2/1 -> MATLAB Function/3(W2)
  Constant/1 -> MATLAB Function/4(Pf)
  Constant1/1 -> MATLAB Function/5(cap_bar)
  MATLAB Function/1(lambda_0) -> lambda_0/1
  M_bar/1 -> MATLAB Function/6(M_bar)

== system predictive_continuous_simulation_20241118_2015b/Predictive_controller1/Predictive input/Subsystem ==
  ym_tf : Inport
  W1 : Inport  Port=2
  W2 : Inport  Port=3
  M_bar : Inport  Port=4
  Constant : Constant  Value=Pf
  Constant1 : Constant  Value=cap_bar
  MATLAB Function : MATLAB Function  TreatAsAtomicUnit=on
  lambda_0 : Outport
  wires:
  ym_tf/1 -> MATLAB Function/1(ym_tf)
  W1/1 -> MATLAB Function/2(W1)
  W2/1 -> MATLAB Function/3(W2)
  Constant/1 -> MATLAB Function/4(Pf)
  Constant1/1 -> MATLAB Function/5(cap_bar)
  MATLAB Function/1(lambda_0) -> lambda_0/1
  M_bar/1 -> MATLAB Function/6(M_bar)

== matlab function predictive_continuous_simulation_20241118_2015b/Subsystem/in_out4 ==
  data: setpoint output; t input; setpoint_vec input; t_num output; setpoint_time input; count input
function [setpoint,t_num]  = fcn(t,setpoint_vec,setpoint_time,count)
%#codegen
%%% 目標値の生成

count_n = count;

if(count_n<=length(setpoint_time) && t>=setpoint_time(int8(count_n)) && t~=0)
    count_n = count_n+1;
end

setpoint = setpoint_vec(int8(count_n));

t_num = count_n;

== matlab function predictive_continuous_simulation_20241118_2015b/Predictive_controller/Predictive input/Subsystem/MATLAB Function ==
  data: ym_tf input; W1 input; W2 input; lambda_0 output; Pf input; cap_bar input; M_bar input
function lambda_0  = fcn(ym_tf,W1,W2,Pf,cap_bar,M_bar)
%#codegen
Wq=ones(4,1);
Wq=W1;

%%% [λ(t0) ν_f]^T の計算
    lambda_nu = M_bar*[Pf*Wq-W2;ym_tf-cap_bar.'*Wq];

    
    lambda_0 = lambda_nu(1:length(lambda_nu)-1,1);  % λ(t0)
%     nu = lambda_nu(length(lambda_nu),:);            % ν_f

== matlab function predictive_continuous_simulation_20241118_2015b/Predictive_controller/Predictive input/in_out ==
  data: ym_vec input; ym_tf output; Tf_n input
function ym_tf = fcn(ym_vec,Tf_n)

% nym=zeros(Tf_n+1,1);
% nym=ym_vec;
%#codegen
ym_tf = ym_vec(1,Tf_n+1);
% ym_tf = nym(Tf_n+1,1);

== matlab function predictive_continuous_simulation_20241118_2015b/ym_sin/MATLAB Function ==
  data: Tf_n_vec input; ym output; t input; Ts input; omega_sin input
function ym = fcn(Tf_n_vec,t,Ts,omega_sin)
a = length(Tf_n_vec)+1

ym = zeros(1,a)
for i = 1:a
    ym(i) = sin(2*pi*omega_sin*(t+(i-1)*Ts))+0.5;
end

== matlab function predictive_continuous_simulation_20241118_2015b/Predictive_controller/Subsystem/MATLAB Function1 ==
  data: ym input; ep input; z2_hat input; a1_vec output; a2_vec output; cap_bar input; beta0 input; Tf_n input; Ts input; Tf input; tstf_vec input; As parameter; exp_cap2 parameter
function [a1_vec,a2_vec] = fcn(ym,ep,z2_hat,cap_bar,beta0,Tf_n,Ts,Tf,tstf_vec,As,exp_cap2)
%#codegen
% % aa,ba,Afp,bfp,r,Pf
%     Aap_bar = [aa zeros(1,length(Afp)); zeros(length(Afp),1) Afp];
%     bap_bar = [ba;bfp];
%     As = [Aap_bar -bap_bar*bap_bar.'/r; -cap_bar*cap_bar.' -Aap_bar.'];
%     
%     M = expm(As*(Tf));                    
%     M1 = M(1:length(M)/2 , 1:length(M)/2);
%     M2 = M(1:length(M)/2 , length(M)/2+1:length(M));
%     M3 = M(length(M)/2+1:length(M) , 1:length(M)/2);
%     M4 = M(length(M)/2+1:length(M) , length(M)/2+1:length(M));
%     
%     M_bar = inv([M4-Pf*M2 -cap_bar; cap_bar.'*M2 0]);
%     
%     bap_v = -bap_bar.'/r;     % ****** %

 %%%--------------------------------------------------------------------%%
 %%%--------------------------------------------------------------------%%
 
a_vec = zeros(length(cap_bar)*2,length(tstf_vec));
a_vec_int = zeros(length(cap_bar)*2,1);

%%%  tf-t0
%%% ∫     exp(As*tau)*tr([0 ca_bar])*ym(tf-tau)*dtau
%%%  0
%%% 台形積分を使用
%%% サンプリング時間ごとの，0からtf-t0までの被積分関数値を計算 
    ii=1;
    for i = 0:Ts:Tf
%         a_vec(:,round(1+i/Ts)) = expm(As*i)*[[1;zeros(length(cap_bar)-1,1)] zeros(length(cap_bar),1); zeros(length(cap_bar),1) cap_bar]*[z2_hat-beta0*ep;ym(round(Tf_n+1-i/Ts))]; 
        a_vec(:,round(1+i/Ts)) = exp_cap2(:,:,ii)*[z2_hat-beta0*ep;ym(round(Tf_n+1-i/Ts))];
%         a_vec(:,round(1+i/Ts)) = exp_cap2(:,:,ii)*[z2_hat;ym(1,round(Tf_n+1-i/Ts))];
        ii=ii+1;
    end
%%% 台形積分
    for i = 1:length(As)
        a_vec_int(i,1) = trapz(tstf_vec,a_vec(i,:));
    end

        a1_vec = a_vec_int(1:length(cap_bar));
        a2_vec = a_vec_int(length(cap_bar)+1:length(cap_bar)*2);

== matlab function predictive_continuous_simulation_20241118_2015b/future signal/MATLAB Function ==
  data: u input; Tf_n_vec input; ym output; u_in input
function ym = fcn(u,Tf_n_vec,u_in)


a = length(Tf_n_vec);
ym = zeros(1,a + 1);
ym(1,1:a) = u_in(1,2:a+1);
ym(1,a+1) = u;

== matlab function predictive_continuous_simulation_20241118_2015b/Subsystem/in_out5 ==
  data: setpoint input; Tref input; Tf_n_vec input; Ts input; ym_out output; ym1 input; ym_in output
function [ym_out,ym_in]   = fcn(setpoint,Tref,Tf_n_vec,Ts,ym1)
%#codegen
%%% 規範信号の生成
%%% 現時刻:ym(t) から 現時刻＋予測時間:ym(t+Tf) まで

nym = length(Tf_n_vec)+1;

ym = zeros(1,nym);
ym(1) = ym1;
    for k = 2:nym
        ym(1,k) = setpoint - exp(-Ts/Tref)*(setpoint-ym(1,k-1));
    end
ym_out = ym;
ym_in = ym(2);

== matlab function predictive_continuous_simulation_20241118_2015b/in_out1 ==
  data: in input; out output
function out = fcn(in)
%#codegen
out = in(1,1);

== matlab function predictive_continuous_simulation_20241118_2015b/Predictive_controller/Subsystem3/MATLAB Function1 ==
  data: ym input; ep input; z2_hat input; v output; cap_bar input; beta0 input; Tf_n input; Ts input; Tf input; tstf_vec input; lamuda_0 input; x_ap input; M3_v_2 parameter; M4_v_2 parameter; As parameter; bap_v parameter; T parameter; exp_cap2 parameter
function v = fcn(ym,ep,z2_hat,cap_bar,beta0,Tf_n,Ts,Tf,tstf_vec,lamuda_0,x_ap,M3_v_2, M4_v_2,As,bap_v,T,exp_cap2)
%#codegen
% aa,ba,Afp,bfp,r,Pf,T
%     Aap_bar = [aa zeros(1,length(Afp)); zeros(length(Afp),1) Afp];
%     bap_bar = [ba;bfp];
%     As = [Aap_bar -bap_bar*bap_bar.'/r; -cap_bar*cap_bar.' -Aap_bar.'];
% 
% M3_v = zeros(length(As)/2,length(As)/2,length(tstf_vec));
% M4_v = zeros(length(As)/2,length(As)/2,length(tstf_vec));
%   for j = 0:Ts:Tf 
%     M = expm(As*(j));                    
% %     M1 = M(1:length(M)/2 , 1:length(M)/2);
% %     M2 = M(1:length(M)/2 , length(M)/2+1:length(M));
%     M3 = M(length(M)/2+1:length(M) , 1:length(M)/2);
%     M4 = M(length(M)/2+1:length(M) , length(M)/2+1:length(M));
%     
%     M3_v(:,:,round(1+j/Ts)) = M3;
%     M4_v(:,:,round(1+j/Ts)) = M4;
%     
%     % M_bar = inv([M4-Pf*M2 -cap_bar; cap_bar.'*M2 0]);  
%     
%         
%   end
%   bap_v = -bap_bar.'/r; 
 %%%--------------------------------------------------------------------%%
 %%%--------------------------------------------------------------------%%
 
a_vec = zeros(length(cap_bar)*2,length(tstf_vec));
a_vec_int = zeros(length(cap_bar)*2,1);

%%%  tf-t0
%%% ∫     exp(As*tau)*tr([0 ca_bar])*ym(tf-tau)*dtau
%%%  0
%%% 台形積分を使用
%%% サンプリング時間ごとの，0からt-t0までの被積分関数値を計算 
a2_vec = zeros(length(cap_bar),length(tstf_vec));
    ii=1;
    for i = 0:Ts:Tf
%         a_vec(:,round(1+i/Ts)) = exp_cap2(:,:,ii)*[z2_hat;ym(round(Tf_n+1-i/Ts))]; 
        a_vec(:,round(1+i/Ts)) = exp_cap2(:,:,ii)*[z2_hat-beta0*ep;ym(round(Tf_n+1-i/Ts))];
        ii=ii+1;
    end
%%% 台形積分
    for i = 1:length(As)
        a_vec_int(i,1) = trapz(tstf_vec,a_vec(i,:));
    end
   for j = 0:Ts:Tf           % j が時刻 t 
%     for i = 0:Ts:j
%         a_vec(:,round(1+i/Ts)) = expm(As*i)*[[1;zeros(length(cap_bar)-1,1)] zeros(length(cap_bar),1); zeros(length(cap_bar),1) cap_bar]*[z2_hat-beta0*ep;ym(round(Tf_n+1-i/Ts))]; 
%     end
% %%% 台形積分
%     for i = 1:length(As)
%         a_vec_int(i,1) = trapz(tstf_vec,a_vec(i,:));
%     end
   
        % a1_vec = a_vec_int(1:length(cap_bar));
        a2_vec(:,round(1+j/Ts)) = a_vec_int(length(cap_bar)+1:length(cap_bar)*2);
   end
 %%%--------------------------------------------------------------------%%
 %%%--------------------------------------------------------------------%%

   v_bar = zeros(1,Tf/Ts+1); % 1+Tf/Ts
    for j = 0:Ts:Tf
     lamuda = M3_v_2(:,:,round(1+j/Ts))*x_ap + M4_v_2(:,:,round(1+j/Ts))*lamuda_0 + a2_vec(:,round(1+j/Ts));
     v_bar(1,round(1+j/Ts)) = bap_v*lamuda;
    end
    
%      v = v_bar(1:round(1+T/Ts));  %%%
   
     v = v_bar(1+T/Ts);  % T/Ts

== matlab function predictive_continuous_simulation_20241118_2015b/Predictive_controller/Predictive input/in_out1 ==
  data: ym_vec input; ym_tf output; Tf_n input
function ym_tf = fcn(ym_vec,Tf_n)

% nym=zeros(Tf_n+1,1);
% nym=ym_vec;
%#codegen
ym_tf = ym_vec(1,Tf_n+1);
% ym_tf = nym(Tf_n+1,1);

== matlab function predictive_continuous_simulation_20241118_2015b/Subsystem1/in_out4 ==
  data: setpoint output; t input; setpoint_vec input; t_num output; setpoint_time input; count input
function [setpoint,t_num]  = fcn(t,setpoint_vec,setpoint_time,count)
%#codegen
%%% 目標値の生成

count_n = count;

if(count_n<=length(setpoint_time) && t>=setpoint_time(int8(count_n)) && t~=0)
    count_n = count_n+1;
end

setpoint = setpoint_vec(int8(count_n));

t_num = count_n;

== matlab function predictive_continuous_simulation_20241118_2015b/Subsystem1/in_out5 ==
  data: setpoint input; Tref input; Tf_n_vec input; Ts input; ym_out output; ym1 input; ym_in output
function [ym_out,ym_in]   = fcn(setpoint,Tref,Tf_n_vec,Ts,ym1)
%#codegen
%%% 規範信号の生成
%%% 現時刻:ym(t) から 現時刻＋予測時間:ym(t+Tf) まで

nym = length(Tf_n_vec)+1;

ym = zeros(1,nym);
ym(1) = ym1;
    for k = 2:nym
        ym(1,k) = setpoint - exp(-Ts/Tref)*(setpoint-ym(1,k-1));
    end
ym_out = ym;
ym_in = ym(2);

== matlab function predictive_continuous_simulation_20241118_2015b/Predictive_controller1/Predictive input/Subsystem/MATLAB Function ==
  data: ym_tf input; W1 input; W2 input; lambda_0 output; Pf input; cap_bar input; M_bar input
function lambda_0  = fcn(ym_tf,W1,W2,Pf,cap_bar,M_bar)
%#codegen
Wq=ones(4,1);
Wq=W1;

%%% [λ(t0) ν_f]^T の計算
    lambda_nu = M_bar*[Pf*Wq-W2;ym_tf-cap_bar.'*Wq];

    
    lambda_0 = lambda_nu(1:length(lambda_nu)-1,1);  % λ(t0)
%     nu = lambda_nu(length(lambda_nu),:);            % ν_f

== matlab function predictive_continuous_simulation_20241118_2015b/Predictive_controller1/Predictive input/in_out ==
  data: ym_vec input; ym_tf output; Tf_n input
function ym_tf = fcn(ym_vec,Tf_n)

% nym=zeros(Tf_n+1,1);
% nym=ym_vec;
%#codegen
ym_tf = ym_vec(1,Tf_n+1);
% ym_tf = nym(Tf_n+1,1);

== matlab function predictive_continuous_simulation_20241118_2015b/Predictive_controller1/Predictive input/in_out1 ==
  data: ym_vec input; ym_tf output; Tf_n input
function ym_tf = fcn(ym_vec,Tf_n)

% nym=zeros(Tf_n+1,1);
% nym=ym_vec;
%#codegen
ym_tf = ym_vec(1,Tf_n+1);
% ym_tf = nym(Tf_n+1,1);

== matlab function predictive_continuous_simulation_20241118_2015b/Predictive_controller1/Subsystem/MATLAB Function1 ==
  data: ym input; ep input; z2_hat input; a1_vec output; a2_vec output; cap_bar input; beta0 input; Tf_n input; Ts input; Tf input; tstf_vec input; As parameter; exp_cap2 parameter
function [a1_vec,a2_vec] = fcn(ym,ep,z2_hat,cap_bar,beta0,Tf_n,Ts,Tf,tstf_vec,As,exp_cap2)
%#codegen
% % aa,ba,Afp,bfp,r,Pf
%     Aap_bar = [aa zeros(1,length(Afp)); zeros(length(Afp),1) Afp];
%     bap_bar = [ba;bfp];
%     As = [Aap_bar -bap_bar*bap_bar.'/r; -cap_bar*cap_bar.' -Aap_bar.'];
%     
%     M = expm(As*(Tf));                    
%     M1 = M(1:length(M)/2 , 1:length(M)/2);
%     M2 = M(1:length(M)/2 , length(M)/2+1:length(M));
%     M3 = M(length(M)/2+1:length(M) , 1:length(M)/2);
%     M4 = M(length(M)/2+1:length(M) , length(M)/2+1:length(M));
%     
%     M_bar = inv([M4-Pf*M2 -cap_bar; cap_bar.'*M2 0]);
%     
%     bap_v = -bap_bar.'/r;     % ****** %

 %%%--------------------------------------------------------------------%%
 %%%--------------------------------------------------------------------%%
 
a_vec = zeros(length(cap_bar)*2,length(tstf_vec));
a_vec_int = zeros(length(cap_bar)*2,1);

%%%  tf-t0
%%% ∫     exp(As*tau)*tr([0 ca_bar])*ym(tf-tau)*dtau
%%%  0
%%% 台形積分を使用
%%% サンプリング時間ごとの，0からtf-t0までの被積分関数値を計算 
    ii=1;
    for i = 0:Ts:Tf
%         a_vec(:,round(1+i/Ts)) = expm(As*i)*[[1;zeros(length(cap_bar)-1,1)] zeros(length(cap_bar),1); zeros(length(cap_bar),1) cap_bar]*[z2_hat-beta0*ep;ym(round(Tf_n+1-i/Ts))]; 
        a_vec(:,round(1+i/Ts)) = exp_cap2(:,:,ii)*[z2_hat-beta0*ep;ym(round(Tf_n+1-i/Ts))];
%         a_vec(:,round(1+i/Ts)) = exp_cap2(:,:,ii)*[z2_hat;ym(1,round(Tf_n+1-i/Ts))];
        ii=ii+1;
    end
%%% 台形積分
    for i = 1:length(As)
        a_vec_int(i,1) = trapz(tstf_vec,a_vec(i,:));
    end

        a1_vec = a_vec_int(1:length(cap_bar));
        a2_vec = a_vec_int(length(cap_bar)+1:length(cap_bar)*2);
